simulink model "absbreak"  (R2020a)
settings: Solver=ode45  StartTime=0.0  StopTime=25  MaxStep=0.01  RelTol=1e-3  AbsTol=1e-6
values from neighbouring files (symbols this model uses):
  I = 5    [abs.mat]
  Kf = 1    [abs.mat]
  PBmax = 1500    [abs.mat]
  Rr = 1.25    [abs.mat]
  TB = 0.01    [abs.mat]
  v0 = 88    [abs.mat]
settings Model: Creator=Admin  LastModifiedBy=Admin
settings SolverCC: AutoScaleAbsTol=off
settings DataIOCC: SaveOutput=off  SaveTime=off

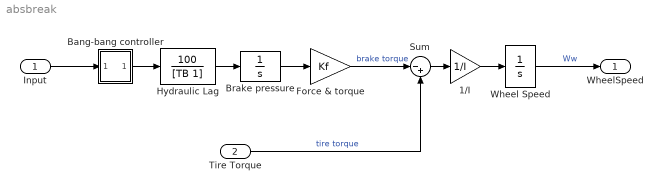
== system absbreak ==
  Input : Inport  OutDataTypeStr=double  PortDimensions=1  SampleTime=0
  Tire Torque : Inport  Port=2  OutDataTypeStr=double  PortDimensions=1  SampleTime=0
  1/I : Gain  Gain=1/I  SaturateOnIntegerOverflow=on  OutDataTypeStr=Inherit: Same as input  ParamDataTypeStr=Inherit: Same as input
  Bang-bang controller : Subsystem  mask(Sign){}
      mask help: y = sign(x)
      mask Help: Sign Function:\n\t\t\ty = 1 if x > 0\n\t\t\ty = 0 if x = 0\n\t\t\ty = -1 if x < 0
      mask Display: plot(-50,-50,50,50,[-50,50],[0,0],[0,0],[-50,50],[-40,0],[-30,-30],[0,40],[30,30])
  Brake pressure : Integrator  LimitOutput=on  UpperSaturationLimit=PBmax  LowerSaturationLimit=0
  Force & torque : Gain  Gain=Kf  SaturateOnIntegerOverflow=on  OutDataTypeStr=Inherit: Same as input  ParamDataTypeStr=Inherit: Same as input
  "Hydraulic Lag " : TransferFcn  Numerator=[100]  Denominator=[TB 1]
  Sum : Sum  Inputs=|-+  InputSameDT=on  SaturateOnIntegerOverflow=on  OutDataTypeStr=Inherit: Same as first input
  Wheel Speed : Integrator  InitialCondition=v0/Rr  LimitOutput=on  UpperSaturationLimit=1000  LowerSaturationLimit=0
  WheelSpeed : Outport  OutDataTypeStr=double  PortDimensions=1  SampleTime=0  VectorParamsAs1DForOutWhenUnconnected=off
  wires:
  Wheel Speed/1 -> WheelSpeed/1  "Ww"
  Brake pressure/1 -> Force & torque/1
  Force & torque/1 -> Sum/1  "brake torque"
  Tire Torque/1 -> Sum/2  "tire torque"
  Bang-bang controller/1(out_1) -> "Hydraulic Lag "/1
  Sum/1 -> 1/I/1
  Input/1 -> Bang-bang controller/1(in_1)
  "Hydraulic Lag "/1 -> Brake pressure/1
  1/I/1 -> Wheel Speed/1

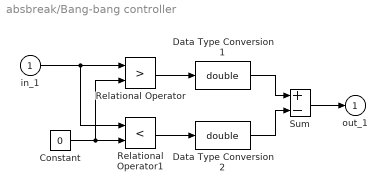
== system absbreak/Bang-bang controller ==
  in_1 : Inport
  Constant : Constant  Value=0
  Data Type Conversion1 : DataTypeConversion  OutDataTypeStr=double  SaturateOnIntegerOverflow=on  RndMeth=Zero
  Data Type Conversion2 : DataTypeConversion  OutDataTypeStr=double  SaturateOnIntegerOverflow=on  RndMeth=Zero
  Relational Operator : RelationalOperator  Operator=>  OutDataTypeStr=boolean  RndMeth=Nearest  InputSameDT=on
  Relational Operator1 : RelationalOperator  Operator=<  OutDataTypeStr=boolean  RndMeth=Nearest  InputSameDT=on
  Sum : Sum  Inputs=+-  InputSameDT=on  SaturateOnIntegerOverflow=on  OutDataTypeStr=Inherit: Same as first input
  out_1 : Outport  InitialOutput=0  VectorParamsAs1DForOutWhenUnconnected=off
  wires:
  in_1/1 -> Relational Operator/1, Relational Operator1/1
  Constant/1 -> Relational Operator1/2, Relational Operator/2
  Relational Operator1/1 -> Data Type Conversion2/1
  Relational Operator/1 -> Data Type Conversion1/1
  Sum/1 -> out_1/1
  Data Type Conversion1/1 -> Sum/1
  Data Type Conversion2/1 -> Sum/2
